simulink model "task5_model"  (R2018a)
settings: Solver=VariableStepAuto  StartTime=0.0  StopTime=20  RelTol=1e-3
values from neighbouring files (symbols this model uses):
  A = [-8.8487+(a-b)/5, -0.0399, -5.55+(c+d)/10, 3.5846 ... (first row only)    [task1.m]    (also in task2.m; task3.m; task4.m; task5.m)
  B = [0.0564+b/(10+c), 0.0319 ... (first row only)    [task1.m]    (also in task2.m; task3.m; task4.m; task5.m)
  C = [-3.2988,-2.1932+(10*c+d)/(100+5*a), 0.0370, -0.0109 ... (first row only)    [task1.m]    (also in task2.m; task3.m; task4.m; task5.m)
  K = Kbar*T    [task1.m]    (also in task2.m = round(((inv(R))*(transpose(B))*P),4); task3.m = round(((inv(R))*(transpose(B))*P),4); task4.m = (inv(Bstar))*Cstarstar; task5.m = round(((inv(R))*(transpose(Bbar))*P),4))
  L = round(transpose(Ktuta),4)    [task3.m]    (also in task5.m)
  X0 = [0.5;-0.1;0.3;-0.8]    [task1.m]    (also in task2.m; task3.m; task4.m; task5.m)
settings Model: Creator=PYT  LastModifiedBy=PYT

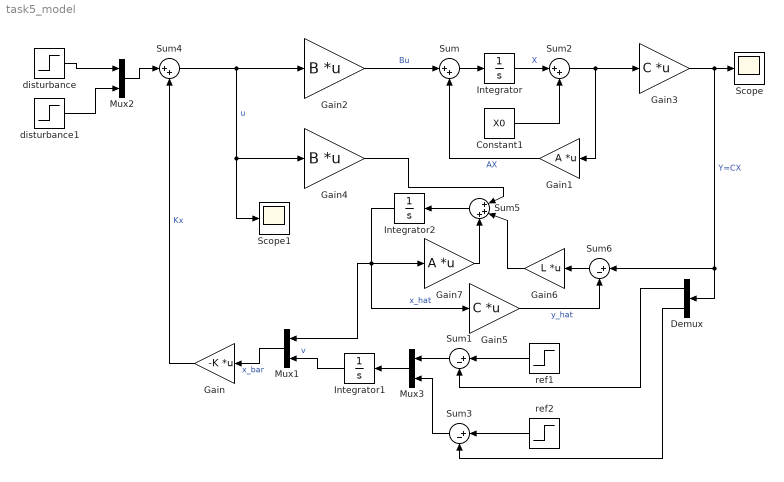
== system task5_model ==
  Constant1 : Constant  Value=X0
  Demux : Demux  Outputs=2
  Gain : Gain  Gain=-K  Multiplication=Matrix(K*u)
  Gain1 : Gain  Gain=A  Multiplication=Matrix(K*u)
  Gain2 : Gain  Gain=B  Multiplication=Matrix(K*u)
  Gain3 : Gain  Gain=C  Multiplication=Matrix(K*u)
  Gain4 : Gain  Gain=B  Multiplication=Matrix(K*u)
  Gain5 : Gain  Gain=C  Multiplication=Matrix(K*u)
  Gain6 : Gain  Gain=L  Multiplication=Matrix(K*u)
  Gain7 : Gain  Gain=A  Multiplication=Matrix(K*u)
  Integrator : Integrator
  Integrator1 : Integrator
  Integrator2 : Integrator
  Mux1 : Mux  Inputs=2
  Mux2 : Mux  Inputs=2
  Mux3 : Mux  Inputs=2
  Scope : Scope
  Scope1 : Scope
  Sum : Sum  Inputs=|++
  Sum1 : Sum  Inputs=|+-
  Sum2 : Sum  Inputs=|++
  Sum3 : Sum  Inputs=|+-
  Sum4 : Sum  Inputs=|++
  Sum5 : Sum  Inputs=|+++
  Sum6 : Sum  Inputs=|+-
  disturbance : Step  Time=10  After=0.3  SampleTime=0
  disturbance1 : Step  Time=10  After=0.2  SampleTime=0
  ref1 : Step  Time=0  After=0.4  SampleTime=0
  ref2 : Step  Time=0  After=0.8  SampleTime=0
  wires:
  Sum/1 -> Integrator/1
  Gain1/1 -> Sum/2  "AX"
  Gain2/1 -> Sum/1  "Bu"
  Gain3/1 -> Sum6/1, Demux/1, Scope/1  "Y=CX"
  Integrator/1 -> Sum2/1  "X"
  Constant1/1 -> Sum2/2
  Sum2/1 -> Gain1/1, Gain3/1
  Mux1/1 -> Gain/1  "x_bar"
  Integrator1/1 -> Mux1/2  "v"
  ref1/1 -> Sum1/1
  disturbance/1 -> Mux2/1
  disturbance1/1 -> Mux2/2
  Demux/1 -> Sum1/2
  Demux/2 -> Sum3/2
  ref2/1 -> Sum3/1
  Mux3/1 -> Integrator1/1
  Sum3/1 -> Mux3/2
  Sum1/1 -> Mux3/1
  Mux2/1 -> Sum4/1
  Sum4/1 -> Gain4/1, Scope1/1, Gain2/1  "u"
  Gain/1 -> Sum4/2  "Kx"
  Gain4/1 -> Sum5/1
  Sum5/1 -> Integrator2/1
  Integrator2/1 -> Mux1/1, Gain7/1, Gain5/1  "x_hat"
  Gain5/1 -> Sum6/2  "y_hat"
  Sum6/1 -> Gain6/1
  Gain6/1 -> Sum5/2
  Gain7/1 -> Sum5/3
